simulink model "Main_Reciever"  (Simulink 8.9)
settings: Solver=VariableStepAuto  StartTime=0.0  StopTime=0.5  RelTol=1e-3
settings Model: Creator=Alam  LastModifiedBy=Alam
settings SolverCC: AutoInsertRateTranBlk=on
settings DataIOCC: SaveFormat=Dataset  SignalLoggingSaveFormat=Dataset  SaveOutput=off  SignalLogging=off  SaveTime=off
settings DebuggingCC: AlgebraicLoopMsg=error  UnderspecifiedInitializationDetection=Simplified  MergeDetectMultiDrivingBlocksExec=error  SingleTaskRateTransMsg=error  FcnCallInpInsideContextMsg=error  AllowSymbolicDim=off  StateNameClashWarn=none
settings HardwareCC: ProdBitPerPointer=64  ProdBitPerSizeT=64  ProdBitPerPtrDiffT=64  ProdLargestAtomicFloat=Float  ProdIntDivRoundTo=Zero  ProdEndianess=LittleEndian  ProdWordSize=64  ProdHWDeviceType=Intel->x86-64 (Windows64)
settings ModelReferenceCC: PropagateSignalLabelsOutOfModel=on
settings GRTTargetCC: CombineOutputUpdateFcns=on  GRTInterface=off
settings ConfigComp: CovMetricSettings=dwe  CovHtmlReporting=off  CovSaveCumulativeToWorkspaceVar=off  CovSaveSingleToWorkspaceVar=off  CovExternalEMLEnable=on

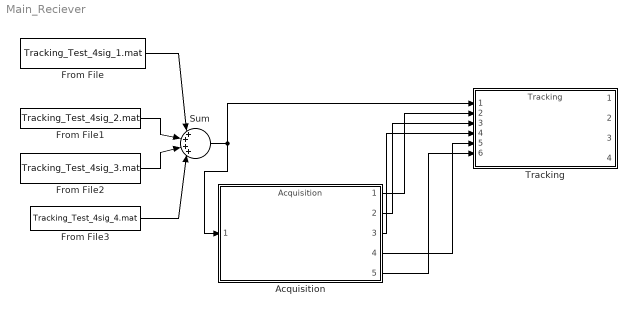
== system Main_Reciever ==
  Acquisition : ModelReference  ModelNameDialog=Acquisition.slx  SimulationMode=Normal  ModelReferenceVersion=1.586
  From File : FromFile  FileName=Tracking_Test_4sig_1.mat  SampleTime=0
  From File1 : FromFile  FileName=Tracking_Test_4sig_2.mat  SampleTime=0
  From File2 : FromFile  FileName=Tracking_Test_4sig_3.mat  SampleTime=0
  From File3 : FromFile  FileName=Tracking_Test_4sig_4.mat  SampleTime=0
  Sum : Sum  Inputs=|++++|
  Tracking : ModelReference  ModelNameDialog=Tracking.slx  SimulationMode=Normal  ModelReferenceVersion=1.592
  wires:
  From File/1 -> Sum/1
  From File1/1 -> Sum/2
  From File3/1 -> Sum/4
  From File2/1 -> Sum/3
  Sum/1 -> Tracking/1, Acquisition/1
  Acquisition/2 -> Tracking/3
  Acquisition/1 -> Tracking/2
  Acquisition/3 -> Tracking/4
  Acquisition/4 -> Tracking/5
  Acquisition/5 -> Tracking/6
